simulink model "Md58StEnCtrl"  (R2018b)
settings: Solver=FixedStepDiscrete  StartTime=0.0  StopTime=10.0  FixedStep=0.01  RelTol=1e-3
undefined symbols (not defined in the file or in its folder): data, KeSMSuFirstRwStBackPosDelta_Val, KeSMSuFirstRwStCushFoldPosDelta_Val, KeSMSuFirstRwStFwdBkwdPosDelta_Val, KeSMSw4SSecRwLtStLgrstOtwdInwdClosePos1_Val, KeSMSw4SSecRwLtStLgrstUpwdDnwdClosePos1_Val, KeSMSw4SSecRwLtStLgrstUpwdDnwdClosePos2_Val, KeSMSw4SSecRwLtStLgrstUpwdDnwdOpenPos1_Val, PassStBkReclnEn_Clear, PassStBkReclnEn_Set, PassStCshnFldEn_Clear, PassStCshnFldEn_Set, PassStFwdBkwdEn_Clear, PassStFwdBkwdEn_Set, SecRwRtStBkReclnEn_Clear, SecRwRtStBkReclnEn_Set, SecRwRtStFwdBkwdEn_Clear, SecRwRtStFwdBkwdEn_Set, SecRwRtStLgrstInwdOtwdEn_Clear, SecRwRtStLgrstInwdOtwdEn_Set, SecRwRtStLgrstUpwdDnwdEn_Clear, SecRwRtStLgrstUpwdDnwdEn_Set, ThdRwLtStBkReclnEn_Clear, ThdRwLtStBkReclnEn_Set, ThdRwLtStFwdBkwdEn_Clear, ThdRwLtStFwdBkwdEn_Set, ThdRwRtStBkReclnEn_Clear, ThdRwRtStBkReclnEn_Set, ThdRwRtStFwdBkwdEn_Clear, ThdRwRtStFwdBkwdEn_Set, ZeroREn_Clear, ZeroREn_Set
libraries: simulink x1
(part 2 of 2)

== system Md58StEnCtrl/Md58StEnCtrl_Cal_sys/Subsystem/If Action Subsystem6 ==
  note: Delete block
  note: Delete block
  Action Port : ActionPort  ActionType=then
  Constant : Constant  Value=21  OutDataTypeStr=uint8
  ThdRwLtStFwdBkwdEn_Set : FunctionCaller  FunctionPrototype=ThdRwLtStFwdBkwdEn_Set(data)  InputArgumentSpecifications=uint8(1)
  wires:
  Constant/1 -> ThdRwLtStFwdBkwdEn_Set/1

== system Md58StEnCtrl/Md58StEnCtrl_Cal_sys/Subsystem/If Action Subsystem7 ==
  Action Port : ActionPort  ActionType=else
  Constant : Constant  Value=21  OutDataTypeStr=uint8
  SecRwRtStLgrstUpwdDnwdEn_Clear : FunctionCaller  FunctionPrototype=SecRwRtStLgrstUpwdDnwdEn_Clear(data)  InputArgumentSpecifications=uint8(1)
  wires:
  Constant/1 -> SecRwRtStLgrstUpwdDnwdEn_Clear/1

== system Md58StEnCtrl/Md58StEnCtrl_Cal_sys/Subsystem/If Action Subsystem8 ==
  Action Port : ActionPort  ActionType=then
  Constant : Constant  Value=21  OutDataTypeStr=uint8
  SecRwRtStLgrstUpwdDnwdEn_Set : FunctionCaller  FunctionPrototype=SecRwRtStLgrstUpwdDnwdEn_Set(data)  InputArgumentSpecifications=uint8(1)
  wires:
  Constant/1 -> SecRwRtStLgrstUpwdDnwdEn_Set/1

== system Md58StEnCtrl/Md58StEnCtrl_Cal_sys/Subsystem/If Action Subsystem9 ==
  Action Port : ActionPort  ActionType=else
  Constant : Constant  Value=21  OutDataTypeStr=uint8
  SecRwRtStLgrstInwdOtwdEn_Clear : FunctionCaller  FunctionPrototype=SecRwRtStLgrstInwdOtwdEn_Clear(data)  InputArgumentSpecifications=uint8(1)
  wires:
  Constant/1 -> SecRwRtStLgrstInwdOtwdEn_Clear/1

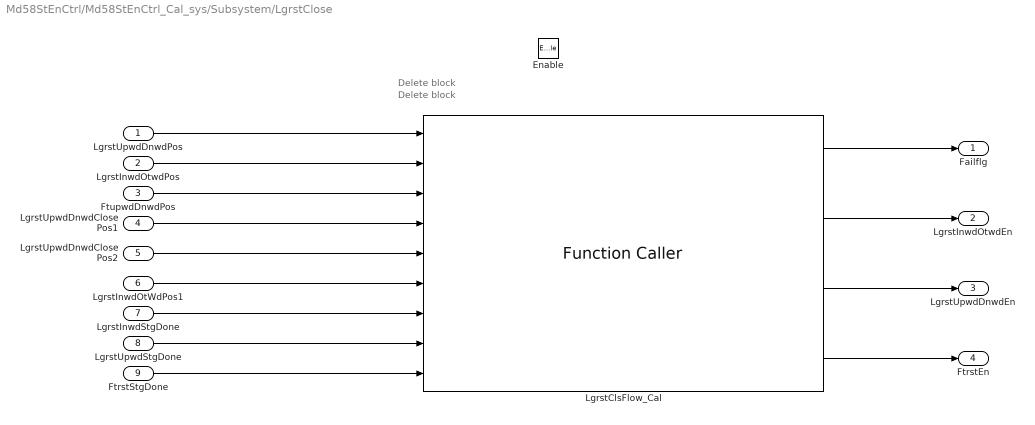
== system Md58StEnCtrl/Md58StEnCtrl_Cal_sys/Subsystem/LgrstClose ==
  note: Delete block
  note: Delete block
  LgrstUpwdDnwdPos : Inport
  LgrstInwdOtwdPos : Inport  Port=2
  FtupwdDnwdPos : Inport  Port=3
  LgrstUpwdDnwdClosePos1 : Inport  Port=4
  LgrstUpwdDnwdClosePos2 : Inport  Port=5
  LgrstInwdOtWdPos1 : Inport  Port=6
  LgrstInwdStgDone : Inport  Port=7
  LgrstUpwdStgDone : Inport  Port=8
  FtrstStgDone : Inport  Port=9
  Enable : EnablePort  StatesWhenEnabling=reset
  LgrstClsFlow_Cal : FunctionCaller  FunctionPrototype=[Failflg,LgrstInwdOtwdEn,LgrstUpwdDnwdEn,FtrstEn] = LgrstClsFlow_Cal(LgrstUpwdDnwdPos,LgrstOtwdInwdPos,FtUpwdDnwdPos,CloseDnwdPos1,CloseDnwdPos2,CloseOtwdPos1,LgrstInwdStgDone,LgrstUpwdStgDone,FtrstStgDone)  InputArgumentSpecifications=uint16(1), uint16(1), uint16(1), uint16(1), uint16(1), uint16(1), boolean(true), boolean(true), boolean(true)  OutputArgumentSpecifications=boolean(true), boolean(true), boolean(true), boolean(true)
  Failflg : Outport
  LgrstInwdOtwdEn : Outport  Port=2
  LgrstUpwdDnwdEn : Outport  Port=3
  FtrstEn : Outport  Port=4
  wires:
  LgrstClsFlow_Cal/1 -> Failflg/1
  LgrstClsFlow_Cal/4 -> FtrstEn/1
  LgrstClsFlow_Cal/3 -> LgrstUpwdDnwdEn/1
  LgrstUpwdDnwdPos/1 -> LgrstClsFlow_Cal/1
  LgrstClsFlow_Cal/2 -> LgrstInwdOtwdEn/1
  LgrstUpwdDnwdClosePos1/1 -> LgrstClsFlow_Cal/4
  LgrstUpwdStgDone/1 -> LgrstClsFlow_Cal/8
  LgrstInwdStgDone/1 -> LgrstClsFlow_Cal/7
  FtrstStgDone/1 -> LgrstClsFlow_Cal/9
  LgrstUpwdDnwdClosePos2/1 -> LgrstClsFlow_Cal/5
  LgrstInwdOtWdPos1/1 -> LgrstClsFlow_Cal/6
  LgrstInwdOtwdPos/1 -> LgrstClsFlow_Cal/2
  FtupwdDnwdPos/1 -> LgrstClsFlow_Cal/3

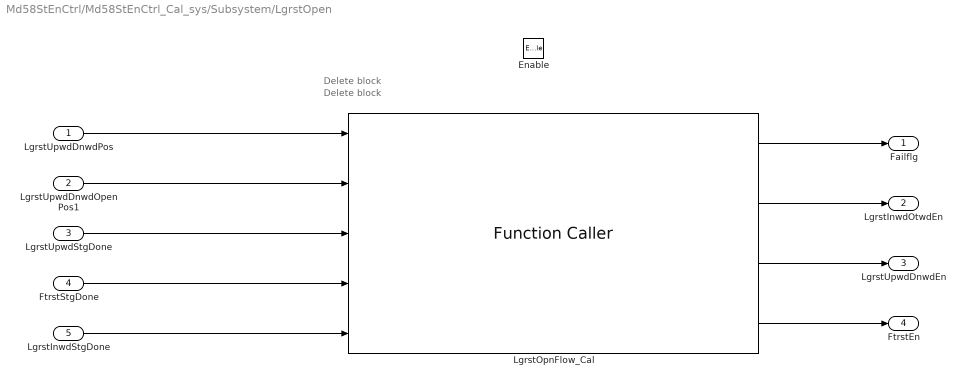
== system Md58StEnCtrl/Md58StEnCtrl_Cal_sys/Subsystem/LgrstOpen ==
  note: Delete block
  note: Delete block
  LgrstUpwdDnwdPos : Inport
  LgrstUpwdDnwdOpenPos1 : Inport  Port=2
  LgrstUpwdStgDone : Inport  Port=3
  FtrstStgDone : Inport  Port=4
  LgrstInwdStgDone : Inport  Port=5
  Enable : EnablePort  StatesWhenEnabling=reset
  LgrstOpnFlow_Cal : FunctionCaller  FunctionPrototype=[Failflg,LgrstInwdOtwdEn,LgrstUpwdDnwdEn,FtrstEn] = LgrstOpnFlow_Cal(LgrstUpwdDnwdPos,LgrstUpwdDnwdOpenPos1,LgrstUpwdStgDone,FtrstStgDone,LgrstInwdStgDone)  InputArgumentSpecifications=uint16(1), uint16(1), boolean(true), boolean(true), boolean(true)  OutputArgumentSpecifications=boolean(true), boolean(true), boolean(true), boolean(true)
  Failflg : Outport
  LgrstInwdOtwdEn : Outport  Port=2
  LgrstUpwdDnwdEn : Outport  Port=3
  FtrstEn : Outport  Port=4
  wires:
  LgrstOpnFlow_Cal/2 -> LgrstInwdOtwdEn/1
  LgrstUpwdDnwdPos/1 -> LgrstOpnFlow_Cal/1
  LgrstOpnFlow_Cal/3 -> LgrstUpwdDnwdEn/1
  FtrstStgDone/1 -> LgrstOpnFlow_Cal/4
  LgrstUpwdStgDone/1 -> LgrstOpnFlow_Cal/3
  LgrstOpnFlow_Cal/4 -> FtrstEn/1
  LgrstInwdStgDone/1 -> LgrstOpnFlow_Cal/5
  LgrstUpwdDnwdOpenPos1/1 -> LgrstOpnFlow_Cal/2
  LgrstOpnFlow_Cal/1 -> Failflg/1

== stateflow chart Md58StEnCtrl/Md58StEnCtrl_Cal_sys/Subsystem/Chart ==
  (default) -> (junction 228) : {
      | ThdRwLtStBkReclnEn = 0;
      | SecRwLtStBkReclnEn = 0;
      | SecRwLtStFrwdBkwdEn = 0;
      | ThdRwLtStFwdBkwdEn = 0;
      | ZeroLEn = 0;
      | LgrstOpnEn = 0;
      | LgrstClsEn = 0;
      | PassStFwdBkwdEn = 0;
      | PassStBkReclnEn = 0;
      | ThdRwRtStBkReclnEn = 0;
      | ThdRwRtStFwdBkwdEn = 0;
      | PassStCshnFldEn = 0;
      | }
  (junction 228) -> (junction 250)
  (junction 250) -> (junction 252) [order 1] : [NotMovPassStFlg ||PassStFwdBkwdStgDone]
  (junction 252) -> (junction 316) [order 1] : [!NotMovPassStFlg&&(PassStFwdBkwdPos<(PassStFwdBkwdTrgtPos1-KeSMSuFirstRwStFwdBkwdPosDelta))&&!PassStBkReclnStgDone]
  (junction 250) -> (junction 258) [order 2] : {PassStFwdBkwdEn = 1;}
  (junction 252) -> (junction 254) [order 2]
  (junction 316) -> (junction 317) : {PassStFwdBkwdFailflg =1;}
  (junction 254) -> (junction 258)
  (junction 317) -> (junction 254)
  (junction 258) -> (junction 273)
  (junction 273) -> (junction 319) [order 1] : [!NotMovPassStFlg]
  (junction 319) -> (junction 331) [order 1] : [PassStFwdBkwdStgDone &&...
      | (PassStFwdBkwdPos>=(PassStFwdBkwdTrgtPos1-KeSMSuFirstRwStFwdBkwdPosDelta)||...
      | PassStBkReclnUpwdDnwdPos>VIPRExitPassStBkReclnUpwdDnwdTrgtPos)]
  (junction 331) -> (junction 334) [order 1] : [PassStBkReclnStgDone ]
  (junction 334) -> (junction 322) [order 1] : [PassStBkReclnUpwdDnwdPos <PassStBkReclnUpwdDnwdTrgtPos1]
  (junction 273) -> (junction 279) [order 2]
  (junction 319) -> (junction 323) [order 2]
  (junction 331) -> (junction 320) [order 2] : {
      | PassStBkReclnEn = 1;
      | }
  (junction 334) -> (junction 335) [order 2]
  (junction 322) -> (junction 324) : {
      | PassStCshnFldFailflg = 1;
      | }
  (junction 335) -> (junction 320)
  (junction 320) -> (junction 333)
  (junction 333) -> (junction 321) [order 1] : [(PassStBkReclnUpwdDnwdPos >=PassStBkReclnUpwdDnwdTrgtPos1)&&...
      | !PassStCshnFldStgDone]
  (junction 333) -> (junction 330) [order 2]
  (junction 321) -> (junction 325) : {PassStCshnFldEn = 1;}
  (junction 323) -> (junction 279)
  (junction 330) -> (junction 323)
  (junction 325) -> (junction 330)
  (junction 324) -> (junction 325)
  (junction 279) -> (junction 234)
  (junction 234) -> (junction 38)
  (junction 38) -> (junction 40) [order 1] : [IfVeSMSuSecRwLtStBkReclnUpwdDnwdPos>VIPLR2LBkReclnUpwdDnwdTrgtPos&&!SecRwLtStBkReclnStgDone]
  (junction 38) -> (junction 44) [order 2]
  (junction 40) -> (junction 42) : {SecRwLtStBkReclnEn = 1;}
  (junction 42) -> (junction 44)
  (junction 44) -> (junction 56)
  (junction 56) -> (junction 58) [order 1] : [LgrstMoveDirection == 1&& !LgrstStgDone]
  (junction 56) -> (junction 62) [order 2]
  (junction 58) -> (junction 60) : {
      | LgrstClsEn = 1;
      | }
  (junction 60) -> (junction 62)
  (junction 62) -> (junction 111)
  (junction 111) -> (junction 113) [order 1] : [IfVeSMSuSecRwLtStZeroPos >VIPLMdR2LZeroTrgtPos && !ZeroLStgDone]
  (junction 111) -> (junction 117) [order 2]
  (junction 113) -> (junction 115) : {ZeroLEn = 1;}
  (junction 115) -> (junction 117)
  (junction 117) -> (junction 147)
  (junction 147) -> (junction 149) [order 1] : [!R3LMdSeatOccupied&&...
      | IfVeSMSuThdRwLtStBkReclnUpwdDnwdPos>VIPRExitR3LBkReclnUpwdDnwdTrgtPos&&...
      | !ThdRwLtStBkReclnStgDone&&...
      | Is7s]
  (junction 147) -> (junction 153) [order 2]
  (junction 149) -> (junction 151) : {
      | ThdRwLtStBkReclnEn = 1;
      | }
  (junction 151) -> (junction 153)
  (junction 153) -> (junction 263)
  (junction 263) -> (junction 266) [order 1] : [!R3RMdSeatOccupied&&...
      | IfVeSMSuThdRwRtStBkReclnUpwdDnwdPos>VIPRExitR3RBkReclnUpwdDnwdTrgtPos&&...
      | !ThdRwRtStBkReclnStgDone]
  (junction 263) -> (junction 270) [order 2]
  (junction 266) -> (junction 268) : {
      | ThdRwRtStBkReclnEn = 1;
      | }
  (junction 268) -> (junction 270)
  (junction 270) -> (junction 65)
  (junction 65) -> (junction 67) [order 1] : [
      | !((IfVeSMSuSecRwLtStBkReclnUpwdDnwdPos<=VIPLR2LBkReclnUpwdDnwdTrgtPos||SecRwLtStBkReclnStgDone)&&...
      | (IfVeSMSuSecRwLtStZeroPos <=VIPLMdR2LZeroTrgtPos ||ZeroLStgDone)&&...
      | (LgrstMoveDirection !=1||LgrstStgDone)&&...
      | (R3LMdSeatOccupied||IfVeSMSuThdRwLtStBkReclnUpwdDnwdPos<=VIPRExitR3LBkReclnUpwdDnwdTrgtPos||ThdRwLtStBkReclnStgDone||!Is7s)&&...
      | (R3RMdSeatOccupied||IfVeSMSuThdRwRtStBkReclnUpwdDnwdPos<=VIPRExitR3RBkReclnUpwdDnwdTrgtPos||ThdRwRtStBkReclnStgDone)&&...
      | PassStDone)
      | ]
  (junction 65) -> (junction 156) [order 2]
  (junction 67) -> (junction 175)
  (junction 156) -> (junction 158) [order 1] : [SecRwLtStFrwdBkwdStgDone]
  (junction 156) -> (junction 162) [order 2] : {SecRwLtStFrwdBkwdEn =1;}
  (junction 158) -> (junction 160)
  (junction 160) -> (junction 162)
  (junction 162) -> (junction 87)
  (junction 87) -> (junction 166) [order 1] : [ThdRwLtStFwdBkwdStgDone||!Is7s]
  (junction 87) -> (junction 170) [order 2] : {ThdRwLtStFwdBkwdEn = 1;}
  (junction 166) -> (junction 168)
  (junction 168) -> (junction 170)
  (junction 170) -> (junction 241)
  (junction 241) -> (junction 243) [order 1] : [ThdRwRtStFwdBkwdStgDone]
  (junction 241) -> (junction 247) [order 2] : {ThdRwRtStFwdBkwdEn = 1;}
  (junction 243) -> (junction 245)
  (junction 245) -> (junction 247)
  (junction 247) -> (junction 173)
  (junction 173) -> (junction 175) [order 1] : [!SecRwLtStFrwdBkwdStgDone||(!ThdRwLtStFwdBkwdStgDone&&Is7s)||...
      | !ThdRwRtStFwdBkwdStgDone]
  (junction 175) -> (junction 177)
  (junction 173) -> (junction 179) [order 2]
  (junction 179) -> (junction 181) [order 1] : [ !ZeroLStgDone]
  (junction 179) -> (junction 185) [order 2]
  (junction 181) -> (junction 183) : {ZeroLEn = 1;}
  (junction 183) -> (junction 185)
  (junction 185) -> (junction 188)
  (junction 188) -> (junction 190) [order 1] : [!SecRwLtStBkReclnStgDone]
  (junction 188) -> (junction 194) [order 2]
  (junction 190) -> (junction 192) : {SecRwLtStBkReclnEn = 1;}
  (junction 192) -> (junction 194)
  (junction 194) -> (junction 282)
  (junction 282) -> (junction 285) [order 1] : [!ThdRwRtStBkReclnStgDone]
  (junction 282) -> (junction 289) [order 2]
  (junction 285) -> (junction 287) : {
      | ThdRwRtStBkReclnEn = 1;
      | }
  (junction 287) -> (junction 289)
  (junction 289) -> (junction 302)
  (junction 302) -> (junction 304) [order 1] : [ThdRwLtStBkReclnStgDone||!Is7s]
  (junction 302) -> (junction 308) [order 2] : {
      | ThdRwLtStBkReclnEn = 1;
      | }
  (junction 304) -> (junction 306)
  (junction 306) -> (junction 308)
  (junction 308) -> (junction 197)
  (junction 197) -> (junction 199) [order 1] : [!LgrstStgDone]
  (junction 197) -> (junction 204) [order 2]
  (junction 199) -> (junction 201) : {LgrstOpnEn = 1;}
  (junction 201) -> (junction 204)
  (junction 177) -> (junction 201)
  (junction 204) -> (junction 261)
  data: IfVeSMSuSecRwLtStBkReclnUpwdDnwdPos input; SecRwLtStBkReclnStgDone input; SecRwLtStFrwdBkwdStgDone input; ThdRwLtStBkReclnStgDone input; ThdRwLtStFwdBkwdStgDone input; VIPLR2LBkReclnUpwdDnwdTrgtPos input; VIPLR2LLgrstUpwdDnwdTrgtPos input; SecRwLtStBkReclnEn output boolean; SecRwLtStFrwdBkwdEn output boolean; ThdRwLtStBkReclnEn output boolean; ThdRwLtStFwdBkwdEn output boolean; ZeroLStgDone input; ZeroLEn output boolean; IfVeSMSuSecRwLtStZeroPos input; VIPLMdR2LZeroTrgtPos input; R3LMdSeatOccupied input; LgrstStgDone input; IfVeSMSuThdRwLtStBkReclnUpwdDnwdPos input; LgrstMoveDirection input uint8 =0; LgrstClsEn output boolean; LgrstOpnEn output boolean; IfVeSMSuThdRwRtStBkReclnUpwdDnwdPos input; NotMovPassStFlg input; R3RMdSeatOccupied input; PassStBkReclnStgDone input; PassStFwdBkwdStgDone input; ThdRwRtStBkReclnStgDone input; ThdRwRtStFwdBkwdStgDone input; VIPRExitR3LBkReclnUpwdDnwdTrgtPos input; VIPRExitR3RBkReclnUpwdDnwdTrgtPos input; ThdRwRtStBkReclnEn output boolean; ThdRwRtStFwdBkwdEn output boolean; PassStFwdBkwdEn output boolean; PassStBkReclnEn output boolean; VIPRExitPassStBkReclnUpwdDnwdTrgtPos input; Is7s input; FirstPassFldFlg input; PassStFldTrgt input; PassStFwdBkwdFailflg output boolean; PassStCshnFldFailflg output boolean; PassStBkReclnUpwdDnwdTrgtPos1 input; PassStFwdBkwdTrgtPos1 input; PassStFwdBkwdPos input; KeSMSuFirstRwStFwdBkwdPosDelta input; PassStCshnFldEn output boolean; PassStCshnFldStgDone input; PassStBkReclnUpwdDnwdPos input; PassStDone input
